simulink model "skynetmini_controller2"  (R2024a)
settings: Solver=FixedStepAuto  StartTime=0.0  StopTime=inf  RelTol=1e-3
libraries: robotlib x5
settings Model: Creator=giorg  LastModifiedBy=Yizhou
settings OptimizationCC: EnhancedBackFolding=on  PassReuseOutputArgsAs=Individual arguments  ZeroExternalMemoryAtStartup=off  ZeroInternalMemoryAtStartup=off  MaxStackSize=64  OptimizeBlockOrder=speed  DifferentSizesBufferReuse=on  OptimizationCustomize=off  EfficientTunableParamExpr=on
settings DebuggingCC: ParameterTunabilityLossMsg=error
settings HardwareCC: ProdBitPerPointer=32  ProdBitPerSizeT=32  ProdBitPerPtrDiffT=32  ProdLargestAtomicFloat=None  ProdIntDivRoundTo=Undefined  ProdEndianess=Unspecified  ProdWordSize=32  ProdHWDeviceType=Generic->Unspecified (assume 32-bit Generic)  UseEmbeddedCoderFeatures=off
settings SFSimCC: MATLABDynamicMemAlloc=off
settings RTWCC: Description=Embedded Coder  SystemTargetFile=ert.tlc  HardwareBoard=Robot Operating System (ROS)  TLCOptions="-aInlineSetEventsForThisBaseRateFcn=TLC_FALSE -aSuppressMultiTaskScheduler=TLC_FALSE  -aRateBasedStepFcn=0"  GenCodeOnly=on  TemplateMakefile=ert_default_tmf  Toolchain=Catkin  TargetLang=C++
settings CodeAppCC: ForceParamTrailComments=on  IgnoreCustomStorageClasses=off  OperatorAnnotations=on  SimulinkDataObjDesc=on  SFDataObjDesc=on  InsertBlockDesc=on
settings ERTTargetCC: SupportNonInlinedSFcns=on

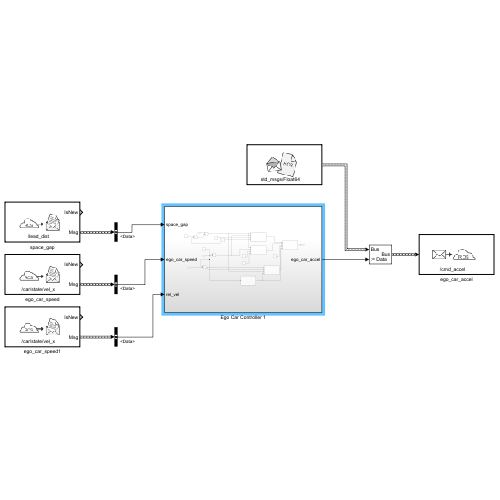
[thumbnail: Simulink's stored preview of the top-level diagram]
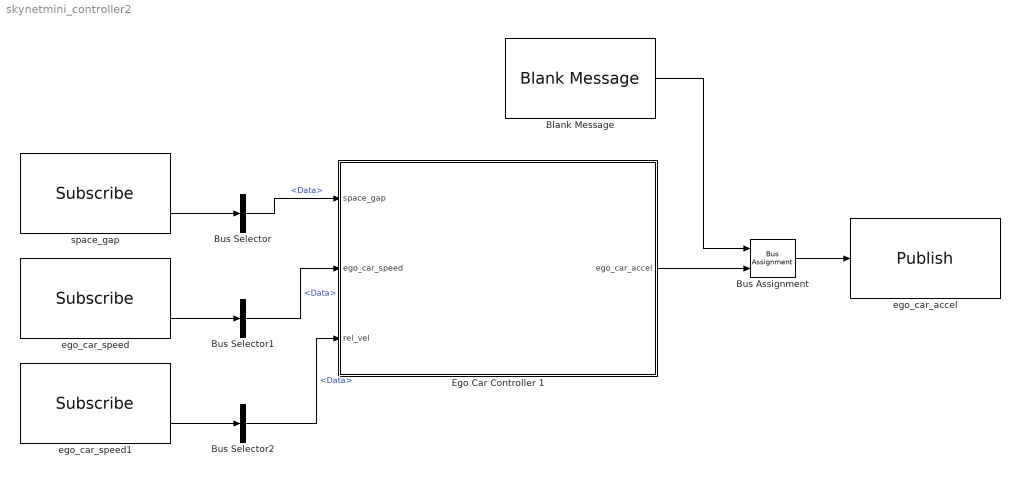
== system skynetmini_controller2 ==
  Blank Message : robotlib/Blank Message  messageClass=Message  entityType=std_msgs/Float64  messageType=std_msgs/Float64  SampleTime=inf  legacyBusStruct=off
  Bus Assignment : BusAssignment  AssignedSignals=Data
  Bus Selector : BusSelector  OutputSignals=Data
  Bus Selector1 : BusSelector  OutputSignals=Data
  Bus Selector2 : BusSelector  OutputSignals=Data
  Ego Car Controller 1 : Subsystem
  ego_car_accel : robotlib/Publish  topicSource=Specify your own  topic=/cmd_accel  messageType=std_msgs/Float64  legacyBusStruct=off  messageQueueLength=1
  ego_car_speed : robotlib/Subscribe  topicSource=Specify your own  topic=/car/state/vel_x  messageType=std_msgs/Float64  SampleTime=-1  legacyBusStruct=off  messageQueueLength=1
  ego_car_speed1 : robotlib/Subscribe  topicSource=Specify your own  topic=/car/state/vel_x  messageType=std_msgs/Float64  SampleTime=-1  legacyBusStruct=off  messageQueueLength=1
  space_gap : robotlib/Subscribe  topicSource=Specify your own  topic=/lead_dist  messageType=std_msgs/Float64  SampleTime=-1  legacyBusStruct=off  messageQueueLength=1
  wires:
  space_gap/2 -> Bus Selector/1
  ego_car_speed/2 -> Bus Selector1/1
  Ego Car Controller 1/1(ego_car_accel) -> Bus Assignment/2
  Bus Selector/1 -> Ego Car Controller 1/1(space_gap)  "<Data>"
  Bus Selector1/1 -> Ego Car Controller 1/2(ego_car_speed)  "<Data>"
  Bus Assignment/1 -> ego_car_accel/1
  Blank Message/1 -> Bus Assignment/1
  Bus Selector2/1 -> Ego Car Controller 1/3(rel_vel)  "<Data>"
  ego_car_speed1/2 -> Bus Selector2/1

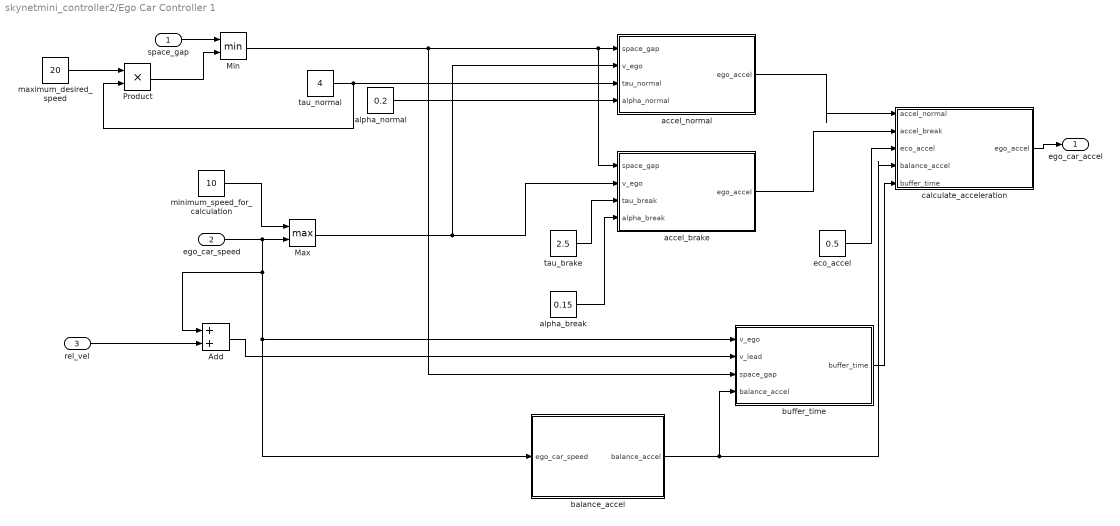
== system skynetmini_controller2/Ego Car Controller 1 ==
  space_gap : Inport
  ego_car_speed : Inport  Port=2
  rel_vel : Inport  Port=3
  Add : Sum
  Max : MinMax  Function=max  Inputs=2
  Min : MinMax  Inputs=2
  Product : Product
  accel_brake : MATLAB Function  TreatAsAtomicUnit=on
  accel_normal : MATLAB Function  TreatAsAtomicUnit=on
  alpha_break : Constant  Value=0.15
  alpha_normal : Constant  Value=0.2
  balance_accel : MATLAB Function  TreatAsAtomicUnit=on
  buffer_time : MATLAB Function  TreatAsAtomicUnit=on
  calculate_acceleration : MATLAB Function  TreatAsAtomicUnit=on
  eco_accel : Constant  Value=0.5
  maximum_desired_speed : Constant  Value=20
  minimum_speed_for_calculation : Constant  Value=10
  tau_brake : Constant  Value=2.5
  tau_normal : Constant  Value=4
  ego_car_accel : Outport
  wires:
  Max/1 -> accel_normal/2(v_ego), accel_brake/2(v_ego)
  Min/1 -> buffer_time/3(space_gap), accel_normal/1(space_gap), accel_brake/1(space_gap)
  alpha_normal/1 -> accel_normal/4(alpha_normal)
  tau_brake/1 -> accel_brake/3(tau_break)
  alpha_break/1 -> accel_brake/4(alpha_break)
  accel_normal/1(ego_accel) -> calculate_acceleration/1(accel_normal)
  eco_accel/1 -> calculate_acceleration/3(eco_accel)
  balance_accel/1(balance_accel) -> buffer_time/4(balance_accel), calculate_acceleration/4(balance_accel)
  accel_brake/1(ego_accel) -> calculate_acceleration/2(accel_break)
  ego_car_speed/1 -> Add/1, buffer_time/1(v_ego), balance_accel/1(ego_car_speed), Max/2
  minimum_speed_for_calculation/1 -> Max/1
  space_gap/1 -> Min/1
  Product/1 -> Min/2
  calculate_acceleration/1(ego_accel) -> ego_car_accel/1
  tau_normal/1 -> Product/2, accel_normal/3(tau_normal)
  maximum_desired_speed/1 -> Product/1
  rel_vel/1 -> Add/2
  buffer_time/1(buffer_time) -> calculate_acceleration/5(buffer_time)
  Add/1 -> buffer_time/2(v_lead)

== matlab function skynetmini_controller2/Ego Car Controller 1/accel_normal ==
  data: space_gap input; v_ego input; tau_normal input; alpha_normal input; ego_accel output
function ego_accel = fcn(space_gap, v_ego, tau_normal, alpha_normal)

ego_accel = (alpha_normal * (space_gap - tau_normal * v_ego));
ego_accel = min(ego_accel, 1.5);
ego_accel = max(ego_accel, -3);

== matlab function skynetmini_controller2/Ego Car Controller 1/accel_brake ==
  data: space_gap input; ego_accel output; v_ego input; tau_break input; alpha_break input
function ego_accel = fcn(space_gap, v_ego, tau_break, alpha_break)

ego_accel = (alpha_break*(space_gap - tau_break * v_ego));
ego_accel = min(ego_accel, 1.5);
ego_accel = max(ego_accel, -3);

== matlab function skynetmini_controller2/Ego Car Controller 1/calculate_acceleration ==
  data: accel_normal input; ego_accel output; accel_break input; eco_accel input; balance_accel input; buffer_time input
function ego_accel = fcn(accel_normal, accel_break, eco_accel, balance_accel, buffer_time) 
    if buffer_time < 10
        ego_accel = min(accel_break,balance_accel);
    elseif accel_normal > 0
        ego_accel = min(accel_normal, eco_accel);
    elseif accel_break > 0
    
        ego_accel = max(accel_normal, balance_accel);
    else
        ego_accel = accel_break;
    end


    if ego_accel > 1.5
        ego_accel = 1.5;
    end
    if ego_accel < -3
        ego_accel = -3;
    end

end

== matlab function skynetmini_controller2/Ego Car Controller 1/balance_accel ==
  data: ego_car_speed input; balance_accel output
function balance_accel = fcn(ego_car_speed)

balance_accel = -0.00021453 * (ego_car_speed * ego_car_speed) - 0.14715;

== matlab function skynetmini_controller2/Ego Car Controller 1/buffer_time ==
  data: v_ego input; v_lead input; space_gap input; buffer_time output; balance_accel input
function buffer_time = fcn(v_ego, v_lead, space_gap, balance_accel)

% Calculate distance needed for ego car to match lead_car speed to brake at
% balance_accel
brake_dist = (v_ego+v_lead)/2*(v_ego - v_lead)/(0-balance_accel);
% Calculate time needed, and safe_dist should be maintained after coasting
buffer_time=(space_gap-brake_dist)/v_ego;
% let maximum speed difference be 3m/s
if (v_ego-v_lead) < 3
    buffer_time = 0;
end
